simulink model "gyro_model"  (R2023a)
settings: Solver=VariableStepAuto  StartTime=0.0  StopTime=100  RelTol=1e-3
undefined symbols (not defined in the file): gyro
libraries: simulink x1
settings Model: Creator=Ameya  LastModifiedBy=Ameya

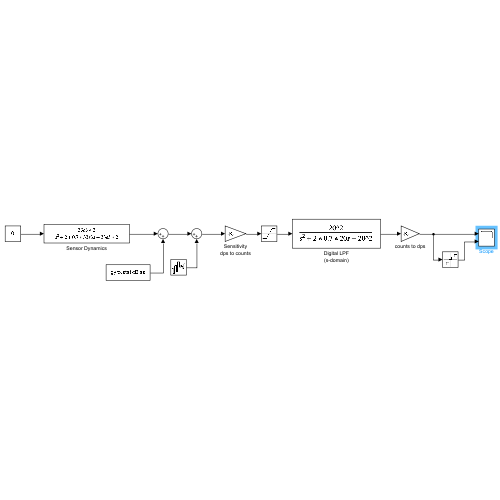
[thumbnail: Simulink's stored preview of the top-level diagram]
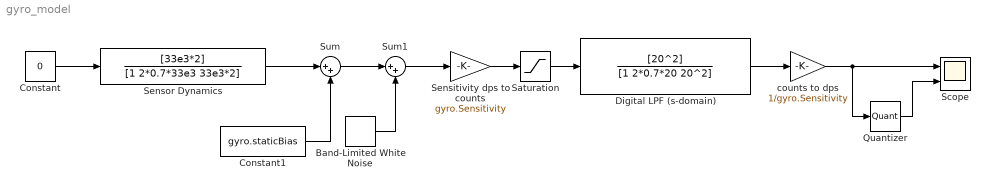
== system gyro_model ==
  Band-Limited White Noise : simulink/Sources/Band-Limited White Noise  Cov=[gyro.NoiseSpectralDensity^2]  Ts=1/10  seed=[23341]
  Constant : Constant  Value=0
  Constant1 : Constant  Value=gyro.staticBias
  Digital LPF (s-domain) : TransferFcn  Numerator=[20^2]  Denominator=[1 2*0.7*20 20^2]
  Quantizer : Quantizer  QuantizationInterval=1/gyro.UpdateRate
  Saturation : Saturate  UpperLimit=+gyro.SatLimit  LowerLimit=-gyro.SatLimit
  Scope : Scope  NumInputPorts=2
  Sensitivity dps to counts : Gain  Gain=gyro.Sensitivity
  Sensor Dynamics : TransferFcn  Numerator=[33e3*2]  Denominator=[1 2*0.7*33e3 33e3*2]
  Sum : Sum  Inputs=|++
  Sum1 : Sum  Inputs=|++
  counts to dps : Gain  Gain=1/gyro.Sensitivity
  wires:
  Constant/1 -> Sensor Dynamics/1
  Constant1/1 -> Sum/2
  Sum/1 -> Sum1/1
  Band-Limited White Noise/1 -> Sum1/2
  Sum1/1 -> Sensitivity dps to counts/1
  Sensitivity dps to counts/1 -> Saturation/1
  Sensor Dynamics/1 -> Sum/1
  Saturation/1 -> Digital LPF (s-domain)/1
  Digital LPF (s-domain)/1 -> counts to dps/1
  counts to dps/1 -> Scope/1, Quantizer/1
  Quantizer/1 -> Scope/2
